simulink model "Inverter_Pulses_Single_Phase"  (R2020a)
settings: Solver=VariableStepAuto  StartTime=0.0  StopTime=3/60  RelTol=1e-3
libraries: powerlib x1
settings Model: Creator=Ricardo Romero  LastModifiedBy=Ricardo Romero

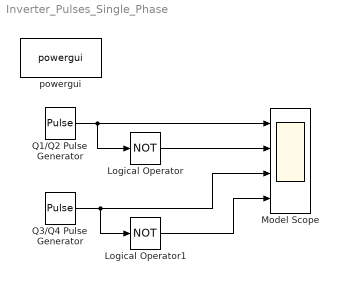
== system Inverter_Pulses_Single_Phase ==
  Logical Operator : Logic  Operator=NOT  AllPortsSameDT=off  OutDataTypeStr=boolean
  Logical Operator1 : Logic  Operator=NOT  AllPortsSameDT=off  OutDataTypeStr=boolean
  Model Scope : Scope  NumInputPorts=4
  Q1/Q2 Pulse Generator : DiscretePulseGenerator  PulseType=Time based  Period=16.66667e-3  PulseWidth=50  PhaseDelay=-1.38889e-3
  Q3/Q4 Pulse Generator : DiscretePulseGenerator  PulseType=Time based  Period=16.66667e-3  PulseWidth=50  PhaseDelay=-6.94444e-3
  powergui : powerlib/powergui  Priority=1  SimulationMode=Continuous  SampleTime=50e-6  frequency=60  Iterations=50  frequencyindice=60  Pbase=100e6  ErrMax=1e-4  UnitsV=kV  UnitsW=MW  buscounter=0  FunctionMessages=off  echomessages=off  EnableUseOfTLC=off  CurrentSourceSwitches=off  DisableSnubberDevices=off  DisableRonSwitches=off  DisableVfSwitches=off  DisplayEquations=off  AutomaticDiscreteSolvers=off  SolverType=Tustin/Backward Euler (TBE)  Interpol=off  ExternalGateDelay=off  methode=off  Ts=100  x0status=blocks  SPID=on  SwTol=0  HookPort=off  NonlinearTolerance=1e-4  nMaxIteration=100  ContinueOnMaxIteration=off  RestoreLinks=warning  ResistiveCurrentMeasurement=off  Frange=[0:2:500]  Ylog=off  Xlog=on  ShowGrid=off  save=off  variable=ZData  structure=0  ZoomFFT=off  StartTime=0.0  cycles=1  DisplayStyle=1  fundamental=60  FreqAxis=off  MaxFrequency=1000  frequencyindicesteady=1  RmsSteady=1  display=off
  wires:
  Q1/Q2 Pulse Generator/1 -> Logical Operator/1, Model Scope/1
  Logical Operator/1 -> Model Scope/2
  Q3/Q4 Pulse Generator/1 -> Logical Operator1/1, Model Scope/3
  Logical Operator1/1 -> Model Scope/4
